simulink model "ex13_4_2"  (Simulink 7.9)
settings: Solver=ode45  StartTime=0.0  StopTime=10.0  RelTol=1e-3
undefined symbols (not defined in the file or in its folder): functieg
settings Model: Creator=Theodor  LastModifiedBy=Theodor
settings DebuggingCC: SolverPrmCheckMsg=none

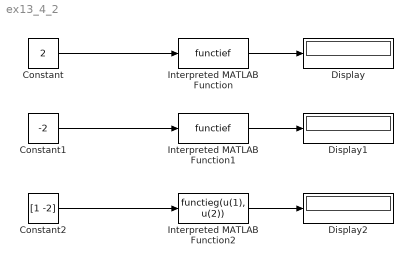
== system ex13_4_2 ==
  Constant : Constant  Value=2
  Constant1 : Constant  Value=-2
  Constant2 : Constant  Value=[1 -2]
  Display : Display
  Display1 : Display
  Display2 : Display
  Interpreted MATLAB Function : MATLABFcn  MATLABFcn=functief
  Interpreted MATLAB Function1 : MATLABFcn  MATLABFcn=functief
  Interpreted MATLAB Function2 : MATLABFcn  MATLABFcn=functieg(u(1), u(2))
  wires:
  Interpreted MATLAB Function/1 -> Display/1
  Constant/1 -> Interpreted MATLAB Function/1
  Interpreted MATLAB Function1/1 -> Display1/1
  Constant1/1 -> Interpreted MATLAB Function1/1
  Interpreted MATLAB Function2/1 -> Display2/1
  Constant2/1 -> Interpreted MATLAB Function2/1
